simulink model "Es6_sim"  (R2017b)
settings: Solver=VariableStepAuto  StartTime=0.0  StopTime=10.0  RelTol=1e-3
values from neighbouring files (symbols this model uses):
  p = 5    [Es6_2.m]
  x0 = [-4 -8]    [Es6_2.m]
settings Model: Creator=claudio  LastModifiedBy=claudio

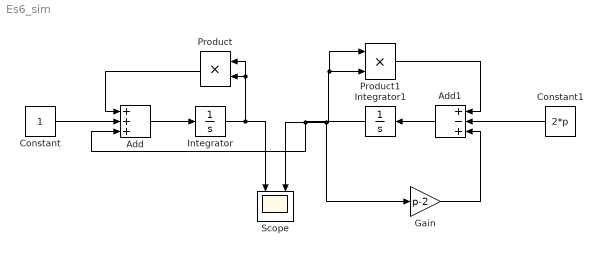
== system Es6_sim ==
  Add : Sum  Inputs=3
  Add1 : Sum  Inputs=+-+
  Constant : Constant
  Constant1 : Constant  Value=2*p
  Gain : Gain  Gain=p-2
  Integrator : Integrator  InitialCondition=x0(1)
  Integrator1 : Integrator  InitialCondition=x0(2)
  Product : Product
  Product1 : Product
  Scope : Scope  NumInputPorts=2
  wires:
  Add/1 -> Integrator/1
  Integrator/1 -> Scope/1, Product/1, Product/2
  Product/1 -> Add/1
  Constant/1 -> Add/2
  Integrator1/1 -> Scope/2, Gain/1, Product1/1, Product1/2, Add/3
  Add1/1 -> Integrator1/1
  Product1/1 -> Add1/1
  Constant1/1 -> Add1/2
  Gain/1 -> Add1/3
